simulink model "modelo_veiculo_7dof"  (R2025a)
settings: Solver=FixedStepAuto  StartTime=0.0  StopTime=10.0  FixedStep=0.001  RelTol=1e-3
undefined symbols (not defined in the file): a, b, C_phi_total, cs, Cy_passive, delta_input, Fz_f_static, Fz_r_static, h_rc, Ix, Iy, Iz, K_phi_f, K_phi_r, K_phi_total, ks, kt, m, ms, mus_q, t_f, t_r, vx
settings Model: Creator=Anderson  LastModifiedBy=Anderson

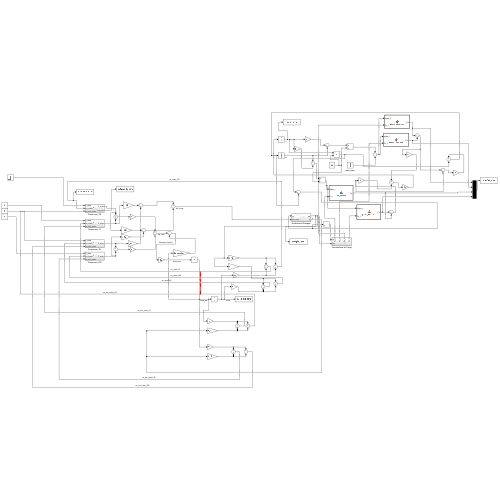
[thumbnail: Simulink's stored preview of the top-level diagram]
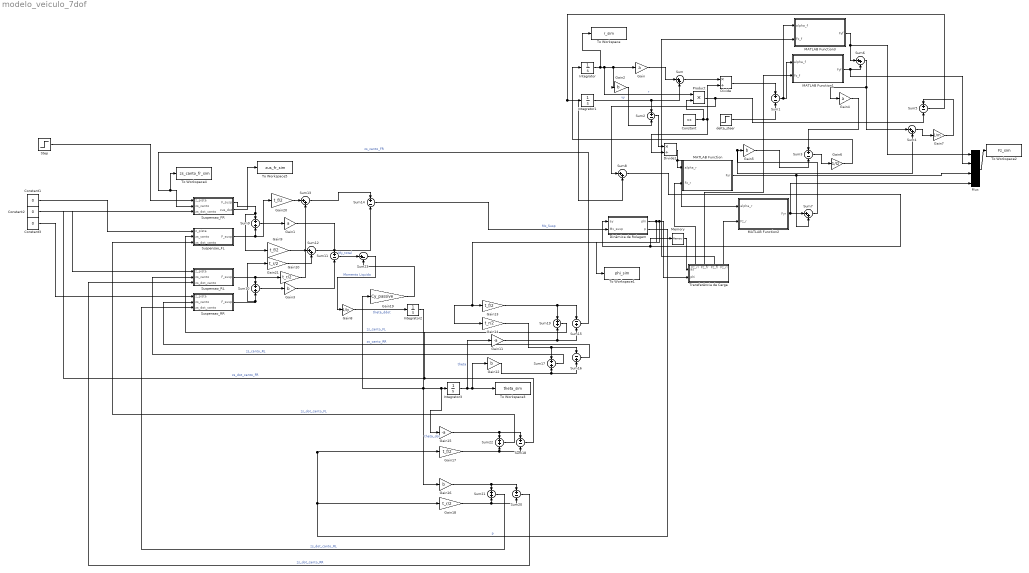
== system modelo_veiculo_7dof ==
  Constant : Constant  Value=vx
  Constant1 : Constant  Value=0
  Constant2 : Constant  Value=0
  Constant3 : Constant  Value=0
  Dinâmica de Rolagem : Subsystem
  Divide : Product  Inputs=*/
  Divide1 : Product  Inputs=*/
  Gain : Gain  Gain=a
  Gain1 : Gain  Gain=a
  Gain{10,14,18,21} (4 alike) : Gain  Gain=t_r/2
  Gain11 : Gain  Gain=-a
  Gain{2..3,5,12,16} (5 alike) : Gain  Gain=b
  Gain{9,13,17,20} (4 alike) : Gain  Gain=t_f/2
  Gain15 : Gain  Gain=-a
  Gain19 : Gain  Gain=Cy_passive
  Gain4 : Gain  Gain=a
  Gain6 : Gain  Gain=1/Iz
  Gain7 : Gain  Gain=1/m
  Gain8 : Gain  Gain=1/Iy
  Integrator{,1..3} (4 alike) : Integrator
  MATLAB Function : MATLAB Function  TreatAsAtomicUnit=on
  MATLAB Function1 : MATLAB Function  TreatAsAtomicUnit=on
  MATLAB Function2 : MATLAB Function  TreatAsAtomicUnit=on
  MATLAB Function3 : MATLAB Function  TreatAsAtomicUnit=on
  Memory : Memory
  Mux : Mux
  Product : Product
  Step : Step  Time=0.5  After=0.1  SampleTime=0
  Sum{,4,6..8,12..13} (7 alike) : Sum  Inputs=|++
  Sum{1..3,5,11,14,18,20} (8 alike) : Sum  Inputs=+-
  Sum{9..10,17,19,21..22} (6 alike) : Sum
  Sum15 : Sum  Inputs=-+
  Sum16 : Sum  Inputs=-+
  Sum23 : Sum  Inputs=|+-
  Suspensao_FL : Subsystem
  Suspensao_FR : Subsystem
  Suspensao_RL : Subsystem
  Suspensao_RR : Subsystem
  To Workspace : ToWorkspace  VariableName=r_sim  SaveFormat=Timeseries  SampleTime=-1
  To Workspace1 : ToWorkspace  VariableName=phi_sim  SaveFormat=Timeseries  SampleTime=-1
  To Workspace2 : ToWorkspace  VariableName=Fz_sim  SaveFormat=Timeseries  SampleTime=-1
  To Workspace3 : ToWorkspace  VariableName=theta_sim  SaveFormat=Timeseries  SampleTime=-1
  To Workspace4 : ToWorkspace  VariableName=zs_canto_fr_sim  SaveFormat=Timeseries  SampleTime=-1
  To Workspace5 : ToWorkspace  VariableName=zus_fr_sim  SaveFormat=Timeseries  SampleTime=-1
  Transferência de Carga : Subsystem
      settings: PortSchema="{\"entries\":[{\"content\":{\"sides\":[{\"content\":{\"connectorIds\":[\"In1\",\"In2\"]},\"type\":\"ConnectorPlacement.EquallySpacedRectSide\",\"uuid\":\"e925ad76-6aec-44f5-ab0f-a760dba7f5fe\"},{\"content\":{\"side\":\"RIGHT\"},\"type\":\"ConnectorPlacement.EquallySpacedRectSide\",\"uuid\":\"3825e0e8-9ec4-4f20-b740-9c23807b7287\"},{\"content\":{\"connectorIds\":[\"Out1\",\"Out2\",\"Out3\",\"Out4\"],\"side\":\"TOP\"},\"type\":\"ConnectorPlacement.EquallySpacedRectSide\",\"uuid\":\"5d8f76d2-4569-4618-8574-d5788c526c3e\"}]},\"type\":\"ConnectorPlacement.EquallySpacedConnector\",\"uuid\":\"9a321bb4-cdbe-47ff-9619-cf02739e8cce\"}],\"packageUris\":[\"http://schema.mathworks.com/mf0/Connector/R2020b\"],\"version\":\"1.0\"}"
  delta_steer : Step  After=delta_input  SampleTime=0
  wires:
  Integrator/1 -> To Workspace/1, Product/1, Gain2/1, Gain/1  "r"
  Integrator1/1 -> Sum2/1, Sum/2  "vy"
  Gain/1 -> Sum/1
  Sum/1 -> Divide/1
  Constant/1 -> Product/2, Divide1/2, Divide/2
  Divide/1 -> Sum1/1
  delta_steer/1 -> Sum1/2
  Sum1/1 -> MATLAB Function3/1(alpha_f), MATLAB Function1/1(alpha_f)
  Gain2/1 -> Sum2/2
  Gain4/1 -> Sum3/1
  Gain5/1 -> Sum3/2
  Sum3/1 -> Gain6/1
  Gain6/1 -> Integrator/1
  Sum4/1 -> Gain7/1
  Gain7/1 -> Sum5/1
  Product/1 -> Sum8/1, Sum5/2
  Sum5/1 -> Sum8/2, Integrator1/1
  Sum2/1 -> Divide1/1
  Divide1/1 -> MATLAB Function2/1(alpha_r), MATLAB Function/1(alpha_r)
  MATLAB Function1/1(Fyf) -> Mux/2, Sum6/2
  Sum6/1 -> Sum4/1, Gain4/1
  MATLAB Function2/1(Fyr) -> Mux/4, Sum7/1
  MATLAB Function/1(Fyr) -> Mux/3, Sum7/2
  Sum7/1 -> Sum4/2, Gain5/1
  Sum8/1 -> Memory/1, Dinâmica de Rolagem/1(ay)
  Dinâmica de Rolagem/1(phi) -> Gain14/1, Gain13/1, To Workspace1/1, Transferência de Carga/2(phi)
  Transferência de Carga/4(Fz_rl) -> MATLAB Function2/2(Fz_r)
  Transferência de Carga/1(Fz_rr) -> MATLAB Function/2(Fz_r)
  Transferência de Carga/2(Fz_fr) -> MATLAB Function1/2(Fz_f)
  Transferência de Carga/3(Fz_fl) -> MATLAB Function3/2(Fz_f)
  MATLAB Function3/1(Fyf) -> Mux/1, Sum6/1
  Mux/1 -> To Workspace2/1
  Memory/1 -> Transferência de Carga/1(ay)
  Gain8/1 -> Integrator2/1  "theta_ddot"
  Integrator2/1 -> Gain15/1, Integrator3/1, Gain19/1, Gain16/1  "theta_dot"
  Integrator3/1 -> Gain11/1, Gain12/1, To Workspace3/1  "theta"
  Sum9/1 -> Gain1/1
  Sum10/1 -> Gain3/1
  Gain1/1 -> Sum11/1
  Gain3/1 -> Sum11/2
  Suspensao_FL/1(F_susp) -> Sum9/2, Gain20/1
  Suspensao_FR/1(F_susp) -> Sum9/1, Gain9/1
  Suspensao_RL/1(F_susp) -> Gain10/1, Sum10/1
  Sum14/1 -> Dinâmica de Rolagem/2(Mx_susp)  "Mx_Susp"
  Gain13/1 -> Sum19/1, Sum15/1
  Gain11/1 -> Sum19/2, Sum15/2
  Sum15/1 -> Suspensao_FR/2(zs_canto), To Workspace4/1  "zs_canto_FR"
  Sum19/1 -> Suspensao_FL/2(zs_canto)  "zs_canto_FL"
  Gain14/1 -> Sum17/1, Sum16/1
  Gain12/1 -> Sum16/2, Sum17/2
  Sum16/1 -> Suspensao_RR/2(zs_canto)  "zs_canto_RR"
  Sum17/1 -> Suspensao_RL/2(zs_canto)  "zs_canto_RL"
  Constant1/1 -> Suspensao_FL/1(z_pista)
  Constant2/1 -> Suspensao_RL/1(z_pista)
  Constant3/1 -> Suspensao_RR/1(z_pista)
  Step/1 -> Suspensao_FR/1(z_pista)
  Dinâmica de Rolagem/2(p) -> Gain18/1, Gain17/1  "p"
  Gain15/1 -> Sum22/1, Sum18/1
  Gain17/1 -> Sum22/2, Sum18/2
  Gain18/1 -> Sum21/2, Sum20/2
  Gain16/1 -> Sum21/1, Sum20/1
  Sum18/1 -> Suspensao_FR/3(zs_dot_canto)  "zs_dot_canto_FR"
  Sum22/1 -> Suspensao_FL/3(zs_dot_canto)  "zs_dot_canto_FL"
  Sum20/1 -> Suspensao_RL/3(zs_dot_canto)  "zs_dot_canto_RR"
  Sum21/1 -> Suspensao_RR/3(zs_dot_canto)  "zs_dot_canto_RL"
  Suspensao_FR/2(zus_dot) -> To Workspace5/1
  Sum11/1 -> Sum23/1  "My_total"
  Gain19/1 -> Sum23/2
  Sum23/1 -> Gain8/1  "Momento Liquido"
  Suspensao_RR/1(F_susp) -> Gain21/1, Sum10/2
  Gain9/1 -> Sum12/1
  Gain21/1 -> Sum12/2
  Gain20/1 -> Sum13/1
  Gain10/1 -> Sum13/2
  Sum13/1 -> Sum14/1
  Sum12/1 -> Sum14/2

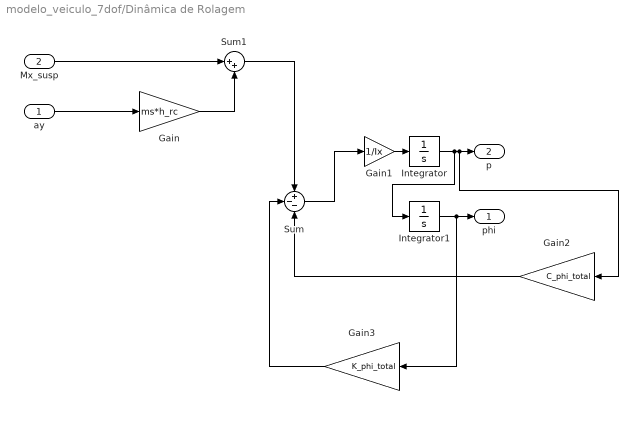
== system modelo_veiculo_7dof/Dinâmica de Rolagem ==
  ay : Inport
  Mx_susp : Inport  Port=2
  Gain : Gain  Gain=ms*h_rc
  Gain1 : Gain  Gain=1/Ix
  Gain2 : Gain  Gain=C_phi_total
  Gain3 : Gain  Gain=K_phi_total
  Integrator : Integrator
  Integrator1 : Integrator
  Sum : Sum  Inputs=+--
  Sum1 : Sum  Inputs=|++
  phi : Outport
  p : Outport  Port=2
  wires:
  ay/1 -> Gain/1
  Gain/1 -> Sum1/2
  Gain1/1 -> Integrator/1
  Integrator/1 -> Integrator1/1, Gain2/1, p/1
  Integrator1/1 -> Gain3/1, phi/1
  Gain3/1 -> Sum/2
  Gain2/1 -> Sum/3
  Mx_susp/1 -> Sum1/1
  Sum1/1 -> Sum/1
  Sum/1 -> Gain1/1

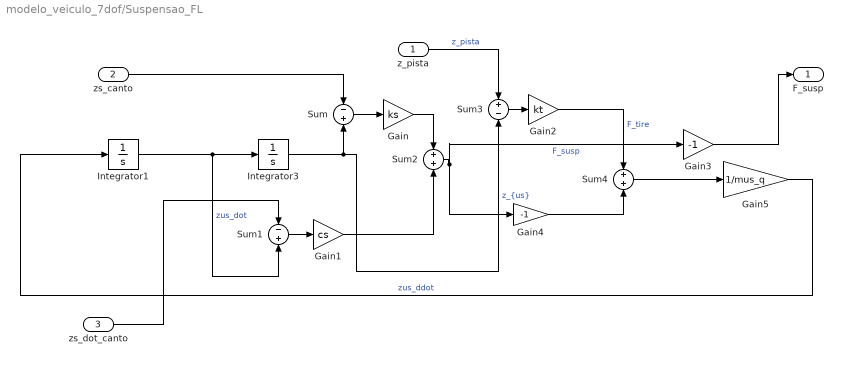
== system modelo_veiculo_7dof/Suspensao_FL ==
  z_pista : Inport
  zs_canto : Inport  Port=2
  zs_dot_canto : Inport  Port=3
  Gain : Gain  Gain=ks
  Gain1 : Gain  Gain=cs
  Gain2 : Gain  Gain=kt
  Gain3 : Gain  Gain=-1
  Gain4 : Gain  Gain=-1
  Gain5 : Gain  Gain=1/mus_q
  Integrator1 : Integrator
  Integrator3 : Integrator
  Sum : Sum  Inputs=-+
  Sum1 : Sum  Inputs=-+
  Sum2 : Sum
  Sum3 : Sum  Inputs=+-
  Sum4 : Sum
  F_susp : Outport
  wires:
  Gain2/1 -> Sum4/1  "F_tire"
  Sum3/1 -> Gain2/1
  Sum2/1 -> Gain3/1, Gain4/1  "F_susp"
  Gain4/1 -> Sum4/2
  z_pista/1 -> Sum3/1  "z_pista"
  Integrator3/1 -> Sum3/2, Sum/2  "z_{us}"
  Sum4/1 -> Gain5/1
  Sum/1 -> Gain/1
  Sum1/1 -> Gain1/1
  Gain5/1 -> Integrator1/1  "zus_ddot"
  Gain1/1 -> Sum2/2
  Gain/1 -> Sum2/1
  Integrator1/1 -> Integrator3/1, Sum1/2  "zus_dot"
  zs_canto/1 -> Sum/1
  zs_dot_canto/1 -> Sum1/1
  Gain3/1 -> F_susp/1

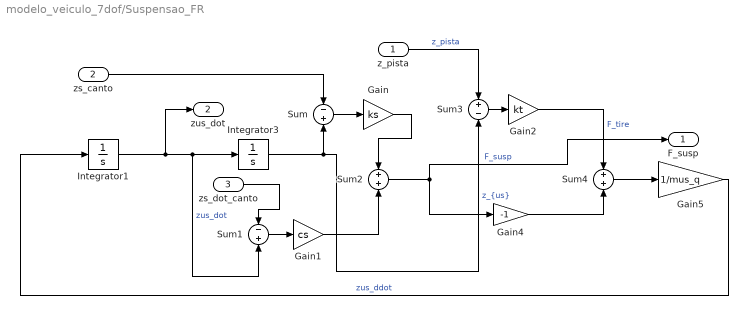
== system modelo_veiculo_7dof/Suspensao_FR ==
  z_pista : Inport
  zs_canto : Inport  Port=2
  zs_dot_canto : Inport  Port=3
  Gain : Gain  Gain=ks
  Gain1 : Gain  Gain=cs
  Gain2 : Gain  Gain=kt
  Gain4 : Gain  Gain=-1
  Gain5 : Gain  Gain=1/mus_q
  Integrator1 : Integrator
  Integrator3 : Integrator
  Sum : Sum  Inputs=-+
  Sum1 : Sum  Inputs=-+
  Sum2 : Sum
  Sum3 : Sum  Inputs=+-
  Sum4 : Sum
  F_susp : Outport
  zus_dot : Outport  Port=2
  wires:
  zs_dot_canto/1 -> Sum1/1
  z_pista/1 -> Sum3/1  "z_pista"
  Sum2/1 -> F_susp/1, Gain4/1  "F_susp"
  Gain2/1 -> Sum4/1  "F_tire"
  Sum3/1 -> Gain2/1
  Integrator1/1 -> zus_dot/1, Integrator3/1, Sum1/2  "zus_dot"
  zs_canto/1 -> Sum/1
  Gain5/1 -> Integrator1/1  "zus_ddot"
  Gain/1 -> Sum2/1
  Gain1/1 -> Sum2/2
  Sum/1 -> Gain/1
  Sum1/1 -> Gain1/1
  Sum4/1 -> Gain5/1
  Integrator3/1 -> Sum3/2, Sum/2  "z_{us}"
  Gain4/1 -> Sum4/2

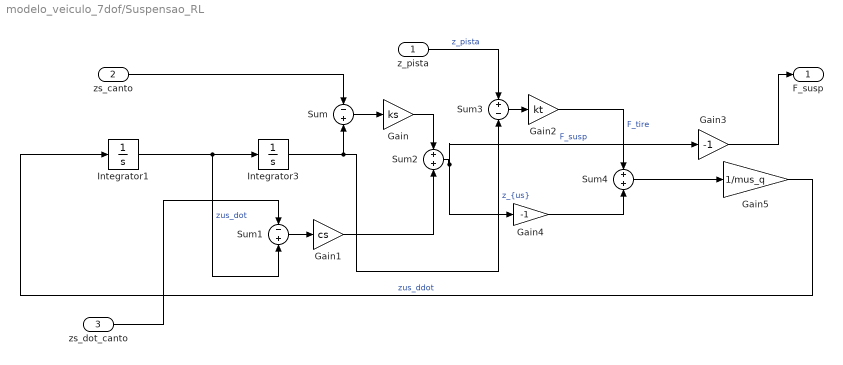
== system modelo_veiculo_7dof/Suspensao_RL ==
  z_pista : Inport
  zs_canto : Inport  Port=2
  zs_dot_canto : Inport  Port=3
  Gain : Gain  Gain=ks
  Gain1 : Gain  Gain=cs
  Gain2 : Gain  Gain=kt
  Gain3 : Gain  Gain=-1
  Gain4 : Gain  Gain=-1
  Gain5 : Gain  Gain=1/mus_q
  Integrator1 : Integrator
  Integrator3 : Integrator
  Sum : Sum  Inputs=-+
  Sum1 : Sum  Inputs=-+
  Sum2 : Sum
  Sum3 : Sum  Inputs=+-
  Sum4 : Sum
  F_susp : Outport
  wires:
  zs_dot_canto/1 -> Sum1/1
  z_pista/1 -> Sum3/1  "z_pista"
  Sum2/1 -> Gain3/1, Gain4/1  "F_susp"
  Gain2/1 -> Sum4/1  "F_tire"
  Sum3/1 -> Gain2/1
  Integrator1/1 -> Integrator3/1, Sum1/2  "zus_dot"
  zs_canto/1 -> Sum/1
  Gain5/1 -> Integrator1/1  "zus_ddot"
  Gain/1 -> Sum2/1
  Gain1/1 -> Sum2/2
  Sum/1 -> Gain/1
  Sum1/1 -> Gain1/1
  Sum4/1 -> Gain5/1
  Integrator3/1 -> Sum3/2, Sum/2  "z_{us}"
  Gain4/1 -> Sum4/2
  Gain3/1 -> F_susp/1

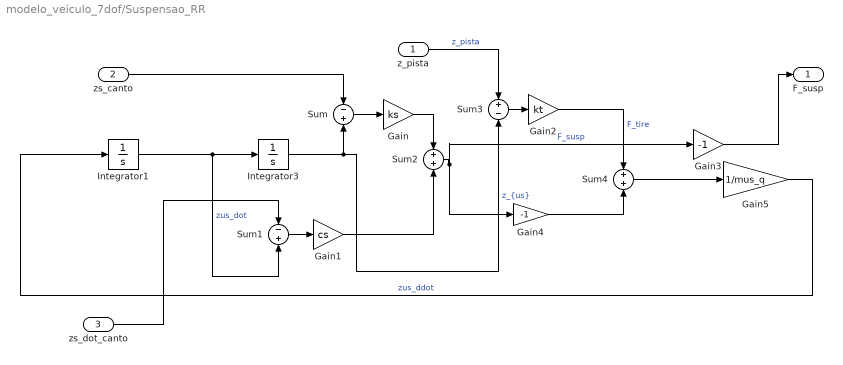
== system modelo_veiculo_7dof/Suspensao_RR ==
  z_pista : Inport
  zs_canto : Inport  Port=2
  zs_dot_canto : Inport  Port=3
  Gain : Gain  Gain=ks
  Gain1 : Gain  Gain=cs
  Gain2 : Gain  Gain=kt
  Gain3 : Gain  Gain=-1
  Gain4 : Gain  Gain=-1
  Gain5 : Gain  Gain=1/mus_q
  Integrator1 : Integrator
  Integrator3 : Integrator
  Sum : Sum  Inputs=-+
  Sum1 : Sum  Inputs=-+
  Sum2 : Sum
  Sum3 : Sum  Inputs=+-
  Sum4 : Sum
  F_susp : Outport
  wires:
  zs_dot_canto/1 -> Sum1/1
  z_pista/1 -> Sum3/1  "z_pista"
  Sum2/1 -> Gain3/1, Gain4/1  "F_susp"
  Gain2/1 -> Sum4/1  "F_tire"
  Sum3/1 -> Gain2/1
  Integrator1/1 -> Integrator3/1, Sum1/2  "zus_dot"
  zs_canto/1 -> Sum/1
  Gain5/1 -> Integrator1/1  "zus_ddot"
  Gain/1 -> Sum2/1
  Gain1/1 -> Sum2/2
  Sum/1 -> Gain/1
  Sum1/1 -> Gain1/1
  Sum4/1 -> Gain5/1
  Integrator3/1 -> Sum3/2, Sum/2  "z_{us}"
  Gain4/1 -> Sum4/2
  Gain3/1 -> F_susp/1

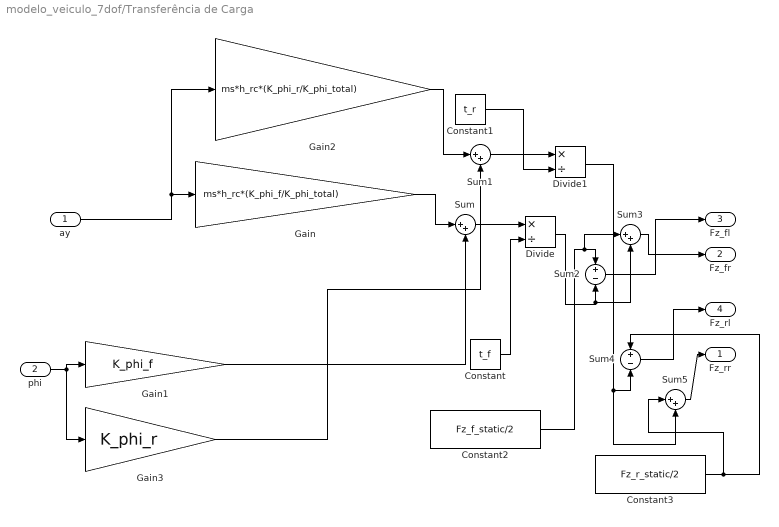
== system modelo_veiculo_7dof/Transferência de Carga ==
  ay : Inport
  phi : Inport  Port=2
  Constant : Constant  Value=t_f
  Constant1 : Constant  Value=t_r
  Constant2 : Constant  Value=Fz_f_static/2
  Constant3 : Constant  Value=Fz_r_static/2
  Divide : Product  Inputs=*/
  Divide1 : Product  Inputs=*/
  Gain : Gain  Gain=ms*h_rc*(K_phi_f/K_phi_total)
  Gain1 : Gain  Gain=K_phi_f
  Gain2 : Gain  Gain=ms*h_rc*(K_phi_r/K_phi_total)
  Gain3 : Gain  Gain=K_phi_r
  Sum{,1,3,5} (4 alike) : Sum  Inputs=|++
  Sum2 : Sum  Inputs=+-
  Sum4 : Sum  Inputs=+-
  Fz_rr : Outport
  Fz_fr : Outport  Port=2
  Fz_fl : Outport  Port=3
  Fz_rl : Outport  Port=4
  wires:
  ay/1 -> Gain2/1, Gain/1
  phi/1 -> Gain3/1, Gain1/1
  Gain/1 -> Sum/1
  Gain1/1 -> Sum/2
  Sum/1 -> Divide/1
  Constant/1 -> Divide/2
  Gain2/1 -> Sum1/1
  Gain3/1 -> Sum1/2
  Constant1/1 -> Divide1/2
  Sum1/1 -> Divide1/1
  Constant2/1 -> Sum3/1, Sum2/1
  Sum2/1 -> Fz_fl/1
  Sum3/1 -> Fz_fr/1
  Divide/1 -> Sum3/2, Sum2/2
  Constant3/1 -> Sum5/1, Sum4/1
  Divide1/1 -> Sum5/2, Sum4/2
  Sum4/1 -> Fz_rl/1
  Sum5/1 -> Fz_rr/1

== matlab function modelo_veiculo_7dof/MATLAB Function ==
  data: alpha_r input; Fyr output; Fz_r input
function Fyr = pneu_traseiro(alpha_r, Fz_r)
% CÓDIGO CORRIGIDO COM INICIALIZAÇÃO

Fyr = 0.0; % <-- ADICIONE ESTA LINHA: Pré-inicializa a variável de saída

% Coeficientes de Pacejka definidos diretamente aqui dentro
B = 10;
C = 1.9;
D_mult = 1.0;
E = 0.97;

% O pico da aderência (D) depende da carga vertical (Fz)
D = D_mult * Fz_r;

% Magic Formula de Pacejka (usando radianos)
phi = (1 - E) * alpha_r + (E / B) * atan(B * alpha_r);
Fyr_mag = D * sin(C * atan(B * phi));

% A força lateral é oposta ao ângulo de deriva
Fyr = -Fyr_mag;

end

== matlab function modelo_veiculo_7dof/MATLAB Function2 ==
  data: alpha_r input; Fyr output; Fz_r input
function Fyr = pneu_traseiro(alpha_r, Fz_r)
% CÓDIGO CORRIGIDO COM INICIALIZAÇÃO

Fyr = 0.0; % <-- ADICIONE ESTA LINHA: Pré-inicializa a variável de saída

% Coeficientes de Pacejka definidos diretamente aqui dentro
B = 10;
C = 1.9;
D_mult = 1.0;
E = 0.97;

% O pico da aderência (D) depende da carga vertical (Fz)
D = D_mult * Fz_r;

% Magic Formula de Pacejka (usando radianos)
phi = (1 - E) * alpha_r + (E / B) * atan(B * alpha_r);
Fyr_mag = D * sin(C * atan(B * phi));

% A força lateral é oposta ao ângulo de deriva
Fyr = -Fyr_mag;

end

== matlab function modelo_veiculo_7dof/MATLAB Function3 ==
  data: alpha_f input; Fyf output; Fz_f input
function Fyf = pneu_dianteiro(alpha_f, Fz_f)
% CÓDIGO CORRIGIDO COM INICIALIZAÇÃO

Fyf = 0.0; % <-- ADICIONE ESTA LINHA: Pré-inicializa a variável de saída

% Coeficientes de Pacejka definidos diretamente aqui dentro
B = 10;
C = 1.9;
D_mult = 1.0;
E = 0.97;

% O pico da aderência (D) depende da carga vertical (Fz)
D = D_mult * Fz_f;

% Magic Formula de Pacejka (usando radianos)
phi = (1 - E) * alpha_f + (E / B) * atan(B * alpha_f);
Fyf_mag = D * sin(C * atan(B * phi));

% A força lateral é oposta ao ângulo de deriva
Fyf = -Fyf_mag;

end

== matlab function modelo_veiculo_7dof/MATLAB Function1 ==
  data: alpha_f input; Fyf output; Fz_f input
function Fyf = pneu_dianteiro(alpha_f, Fz_f)
% CÓDIGO CORRIGIDO COM INICIALIZAÇÃO

Fyf = 0.0; % <-- ADICIONE ESTA LINHA: Pré-inicializa a variável de saída

% Coeficientes de Pacejka definidos diretamente aqui dentro
B = 10;
C = 1.9;
D_mult = 1.0;
E = 0.97;

% O pico da aderência (D) depende da carga vertical (Fz)
D = D_mult * Fz_f;

% Magic Formula de Pacejka (usando radianos)
phi = (1 - E) * alpha_f + (E / B) * atan(B * alpha_f);
Fyf_mag = D * sin(C * atan(B * phi));

% A força lateral é oposta ao ângulo de deriva
Fyf = -Fyf_mag;

end
